simulink model "untitled"  (R2012b)
settings: Solver=ode45  StartTime=0.0  StopTime=6  RelTol=1e-3
undefined symbols (not defined in the file): A, Ahat, B, Bhat, C, L
libraries: simulink x1
settings Model: Creator=Juliano  LastModifiedBy=Juliano

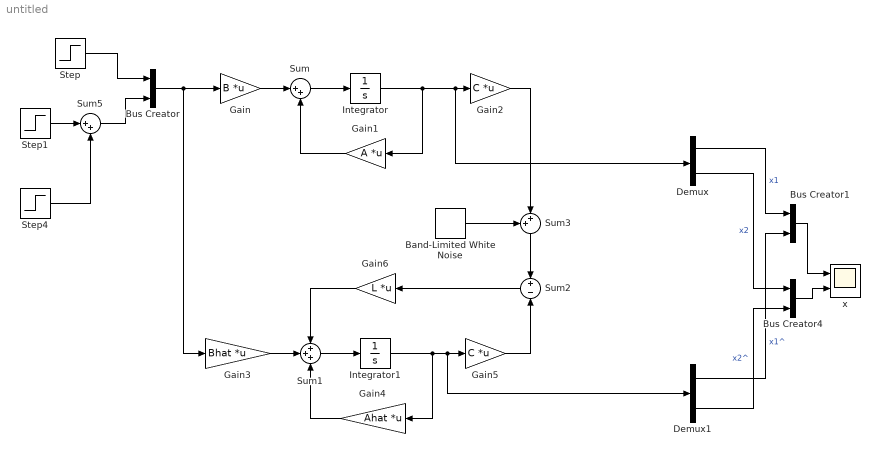
== system untitled ==
  Band-Limited White Noise : simulink/Sources/Band-Limited White Noise  Cov=[0.05]  Ts=0.01  seed=[23341]
  Bus Creator : BusCreator  Inputs=2
  Bus Creator1 : BusCreator  Inputs=2
  Bus Creator4 : BusCreator  Inputs=2
  Demux : Demux  Outputs=2
  Demux1 : Demux  Outputs=2
  Gain : Gain  Gain=B  Multiplication=Matrix(K*u)
  Gain1 : Gain  Gain=A  Multiplication=Matrix(K*u)
  Gain2 : Gain  Gain=C  Multiplication=Matrix(K*u)
  Gain3 : Gain  Gain=Bhat  Multiplication=Matrix(K*u)
  Gain4 : Gain  Gain=Ahat  Multiplication=Matrix(K*u)
  Gain5 : Gain  Gain=C  Multiplication=Matrix(K*u)
  Gain6 : Gain  Gain=L  Multiplication=Matrix(K*u)
  Integrator : Integrator
  Integrator1 : Integrator
  Step : Step  Time=0  SampleTime=0
  Step1 : Step  After=10  SampleTime=0
  Step4 : Step  Time=4  After=-20  SampleTime=0
  Sum : Sum  Inputs=|++
  Sum1 : Sum  Inputs=+++
  Sum2 : Sum  Inputs=+-
  Sum3 : Sum  Inputs=++|
  Sum5 : Sum  Inputs=|++
  x : Scope  NumInputPorts=2
      settings: ShowLegends=on  YMin=-5~-5  YMax=5~5  SaveName=ScopeData2
  wires:
  Step/1 -> Bus Creator/1
  Gain/1 -> Sum/1
  Sum/1 -> Integrator/1
  Gain1/1 -> Sum/2
  Integrator/1 -> Demux/1, Gain2/1, Gain1/1
  Sum1/1 -> Integrator1/1
  Integrator1/1 -> Gain4/1, Demux1/1, Gain5/1
  Gain5/1 -> Sum2/2
  Gain4/1 -> Sum1/3
  Gain3/1 -> Sum1/2
  Sum2/1 -> Gain6/1
  Gain6/1 -> Sum1/1
  Bus Creator/1 -> Gain3/1, Gain/1
  Bus Creator1/1 -> x/1
  Bus Creator4/1 -> x/2
  Demux/1 -> Bus Creator1/1  "x1"
  Demux1/1 -> Bus Creator1/2  "x1^"
  Demux/2 -> Bus Creator4/1  "x2"
  Demux1/2 -> Bus Creator4/2  "x2^"
  Step1/1 -> Sum5/1
  Sum5/1 -> Bus Creator/2
  Step4/1 -> Sum5/2
  Sum3/1 -> Sum2/1
  Gain2/1 -> Sum3/2
  Band-Limited White Noise/1 -> Sum3/1
